simulink model "multi_model1"  (R2016a)
settings: Solver=ode3  SolverMode=SingleTasking  StartTime=0.0  StopTime=inf  FixedStep=0.01  RelTol=1e-3
values from neighbouring files (symbols this model uses):
  s = serial (serPort)    [UART_Connector.m]
undefined symbols (not defined in the file or in its folder): deg, rad
libraries: simulink x19, aerolibconvert2 x2, aerolibobsolete x1, aerolibatmos2 x1, aerolibnav x1, aerolibanimutils x1
(part 2 of 2)

== matlab function multi_model1/Control System/pwm_out ==
  data: Roll input; M1 output; Pitch input; Thrust input; Yaw input; M2 output; M3 output; M4 output; M5 output; M6 output; M7 output; M8 output
function [M1, M2, M3, M4, M5, M6, M7, M8] = motor_mixer(Roll, Pitch, Thrust, Yaw)

%===========================Settings & Constants===========================

idle_PWM = 1122;
aircraft_mixer = 3;
% Quad [X] = 0
% Quad [+] = 1
% Hex  [X] = 2

%===============================Quad X Mixer===============================

if aircraft_mixer == 0;        % Quad X
    M1 = ((Roll + Pitch - Yaw) * Thrust / 2 + Thrust) * 800 + idle_PWM;
    M2 = ((-Roll + Pitch + Yaw) * Thrust / 2 + Thrust) * 800 + idle_PWM;
    M3 = ((-Roll - Pitch - Yaw) * Thrust / 2 + Thrust) * 800 + idle_PWM;
    M4 = ((Roll - Pitch + Yaw) * Thrust / 2 + Thrust) * 800 + idle_PWM;
    M5 = 1122;
    M6 = 1122;
    M7 = 1122;
    M8 = 1122;
elseif aircraft_mixer == 1;    % Quad +
    M1 = ((Pitch - Yaw) * Thrust / 2 + Thrust) * 800 + idle_PWM;
    M2 = ((-Roll + Yaw) * Thrust / 2 + Thrust) * 800 + idle_PWM;
    M3 = ((-Pitch - Yaw) * Thrust / 2 + Thrust) * 800 + idle_PWM;
    M4 = ((Roll + Yaw) * Thrust / 2 + Thrust) * 800 + idle_PWM;
    M5 = 1122;
    M6 = 1122;
    M7 = 1122;
    M8 = 1122;
elseif aircraft_mixer == 2;    % Hex X
    M1 = ((Pitch + Roll / 2 - Yaw) * Thrust / 2 + Thrust) * 800 + idle_PWM;
    M2 = ((Pitch - Roll / 2 + Yaw) * Thrust / 2 + Thrust) * 800 + idle_PWM;
    M3 = ((-Roll - Yaw) * Thrust / 2 + Thrust) * 800 + idle_PWM;
    M4 = ((-Pitch - Roll / 2 + Yaw) * Thrust / 2 + Thrust) * 800 + idle_PWM;
    M5 = ((-Pitch + Roll / 2 - Yaw) * Thrust / 2 + Thrust) * 800 + idle_PWM;
    M6 = ((Roll + Yaw) * Thrust / 2 + Thrust) * 800 + idle_PWM;
    M7 = 1122;
    M8 = 1122;
elseif aircraft_mixer == 3;    % Octa +
    M1 = ((-Pitch - Yaw)* Thrust / 8 + Thrust)* 800 + idle_PWM;    
    M2 = (( Pitch - Yaw)* Thrust / 8 + Thrust)* 800 + idle_PWM;
    M3 = (((-Pitch - Roll)* sqrt(2)/2 + Yaw)* Thrust / 8 + Thrust)* 800 + idle_PWM;    
    M4 = ((( Pitch - Roll)* sqrt(2)/2 + Yaw)* Thrust / 8 + Thrust)* 800 + idle_PWM;    
    M5 = (((-Pitch + Roll)* sqrt(2)/2 + Yaw)* Thrust / 8 + Thrust)* 800 + idle_PWM;    
    M6 = ((( Pitch + Roll)* sqrt(2)/2 + Yaw)* Thrust / 8 + Thrust)* 800 + idle_PWM;    
    M7 = (( Roll - Yaw)* Thrust / 8 + Thrust)* 800 + idle_PWM;
    M8 = ((-Roll - Yaw)* Thrust / 8 + Thrust)* 800 + idle_PWM;
else
    M1 = 1122;
    M2 = 1122;
    M3 = 1122;
    M4 = 1122;
    M5 = 1122;
    M6 = 1122;
    M7 = 1122;
    M8 = 1122;
end
%==========================================================================

== matlab function multi_model1/Signal Receiver/MATLAB Function ==
  data: WPdataTable output
function WPdataTable = getWP()
WPdataTable = [0 0 5; 0 3 5; 4 3 5; 0 0 5; 0 0 2];
